simulink library "coefficientsOfTunableBandpassFilter"  (R2021a)
settings: Solver=VariableStepAuto  StartTime=0.0  StopTime=10.0  RelTol=1e-3
undefined symbols (not defined in the file): centerFrequency, qualityFactor
libraries: simulink x1
Description:
  | These coefficients are for use with the QRS_Detector_Library within the tunableBandpassFilter component.
  | These coefficients complete the difference equation of the tunable bandpass filter.
settings Model: Creator=wallyproenza  LastModifiedBy=wallyproenza

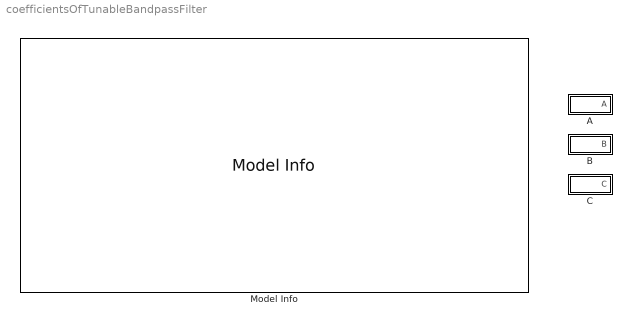
== system coefficientsOfTunableBandpassFilter ==
  A : Subsystem  AncestorBlock=QRS_Detector_Library/tunableBandpassFilter/A
  B : Subsystem  AncestorBlock=QRS_Detector_Library/tunableBandpassFilter/B
  C : Subsystem  AncestorBlock=QRS_Detector_Library/tunableBandpassFilter/C
  Model Info : simulink/Model-Wide Utilities/Model Info  Frame=on  DisplayStringWithTags=|  HorizontalTextAlignment=Center  LeftAlignmentValue=0.5
      | Model Info
      | %<ModelName>
      | 
      | %<Description>

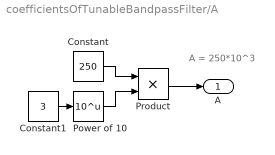
== system coefficientsOfTunableBandpassFilter/A ==
  note: A = 250*10^3
  Constant : Constant  Value=250
  Constant1 : Constant  Value=3
  Power of 10 : Math  Operator=10^u  SaturateOnIntegerOverflow=on
  Product : Product
  A : Outport
  wires:
  Power of 10/1 -> Product/2
  Constant/1 -> Product/1
  Product/1 -> A/1
  Constant1/1 -> Power of 10/1

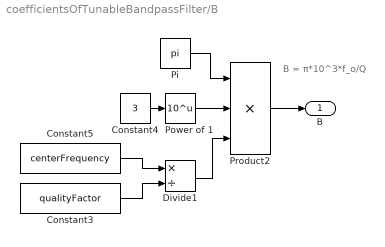
== system coefficientsOfTunableBandpassFilter/B ==
  note: B = π*10^3*f_o/Q
  Constant3 : Constant  Value=qualityFactor
  Constant4 : Constant  Value=3
  Constant5 : Constant  Value=centerFrequency
  Divide1 : Product  Inputs=*/
  Pi : Constant  Value=pi  OutDataTypeStr=Inherit: Inherit via back propagation
  Power of 1 : Math  Operator=10^u  SaturateOnIntegerOverflow=on
  Product2 : Product  Inputs=3
  B : Outport
  wires:
  Product2/1 -> B/1
  Constant5/1 -> Divide1/1
  Divide1/1 -> Product2/3
  Power of 1/1 -> Product2/2
  Constant3/1 -> Divide1/2
  Pi/1 -> Product2/1
  Constant4/1 -> Power of 1/1

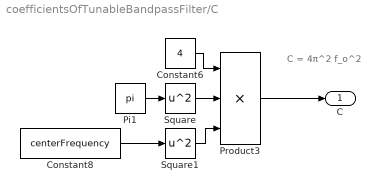
== system coefficientsOfTunableBandpassFilter/C ==
  note: C = 4π^2 f_o^2
  Constant6 : Constant  Value=4
  Constant8 : Constant  Value=centerFrequency
  Pi1 : Constant  Value=pi  OutDataTypeStr=Inherit: Inherit via back propagation
  Product3 : Product  Inputs=3
  Square : Math  Operator=square  SaturateOnIntegerOverflow=on
  Square1 : Math  Operator=square  SaturateOnIntegerOverflow=on
  C : Outport
  wires:
  Product3/1 -> C/1
  Square1/1 -> Product3/3
  Square/1 -> Product3/2
  Pi1/1 -> Square/1
  Constant8/1 -> Square1/1
  Constant6/1 -> Product3/1
